simulink model "baseline1"  (R2022b)
settings: Solver=ode4  StartTime=0.0  StopTime=200  FixedStep=1e-3  RelTol=1e-3
undefined symbols (not defined in the file or in its folder): A_do, B_do, c_uf, do_w, f_b, f_max, f_min, F_TOT_MAX, Fz_min, g, G_do, Gamma_mix, Ixx, Iyy, Izz, K_eta, K_omega, K_w, Ka1, Ka2, Ka3, Kgamma, Knu, Kp1, Kp2, Kp3, L, l_axis, l_gain, m, m_p, n_state_axis, p2_bias_acc, p2_h3_s0, p2_ic_do, p2_ic_eso, p2_ic_pos, p2_ic_vel, p2_nd_pos, p2_prm, p2_prm_h3, p2_prm_m3, p2_prm_n6, p2_prm_w, p2_seed_acc, p2_seed_gyro, p2_seed_pos, p2_tau_m, p2_trim_do, p2_trim_eso, p2_trim_ff_v, p2_Ts_att, p2_Ts_pos, p2_var_acc, p2_var_gyro, p2_var_pos, payload_amp, payload_inj_on, payload_K_ratio, payload_model ... (+18)
(part 1 of 3)
settings Model: Creator=Dell  LastModifiedBy=Dell

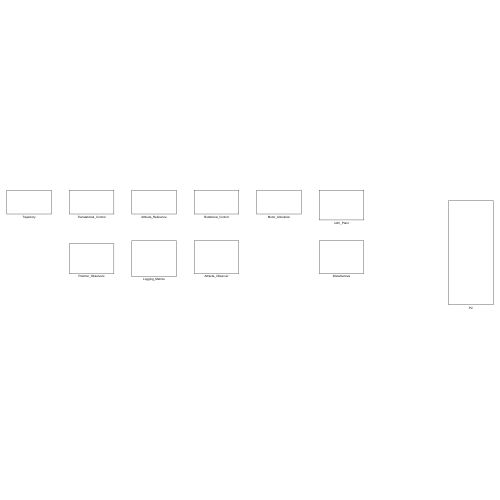
[thumbnail: Simulink's stored preview of the top-level diagram]
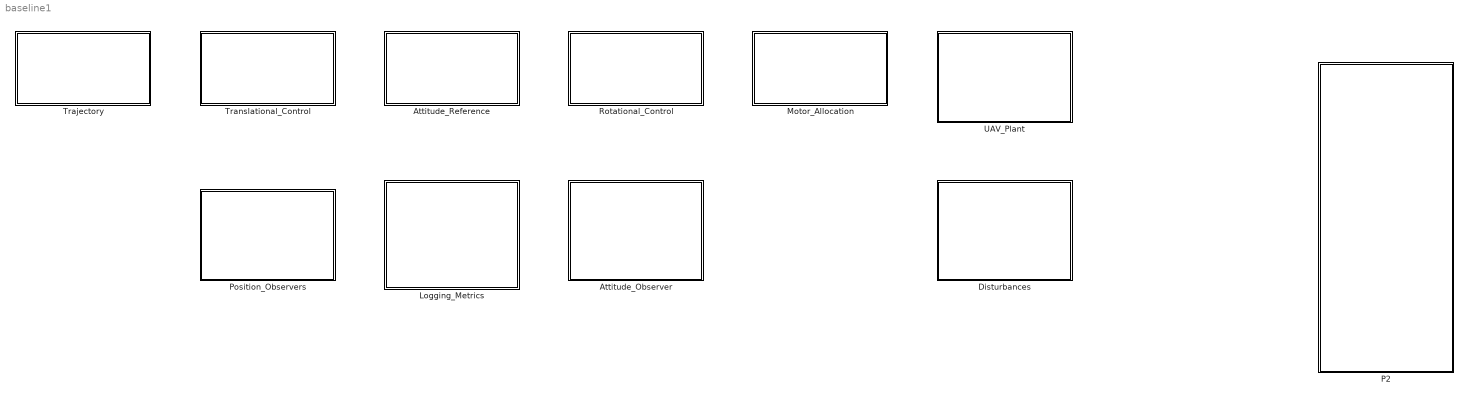
== system baseline1 ==
  Attitude_Observer : Subsystem
  Attitude_Reference : Subsystem
  Disturbances : Subsystem
  Logging_Metrics : Subsystem
  Motor_Allocation : Subsystem
  P2 : Subsystem
  Position_Observers : Subsystem
  Rotational_Control : Subsystem
  Trajectory : Subsystem
  Translational_Control : Subsystem
  UAV_Plant : Subsystem

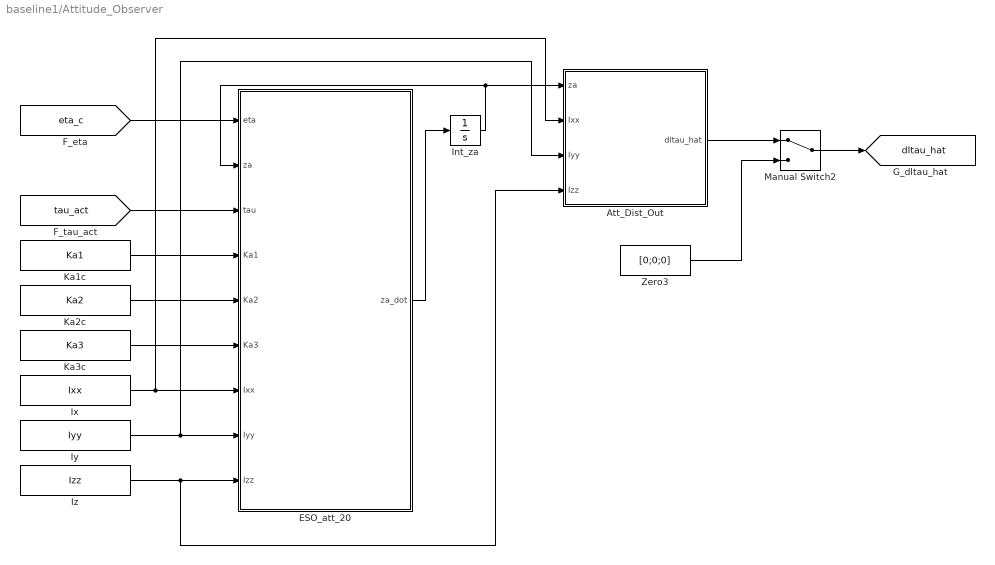
== system baseline1/Attitude_Observer ==
  Att_Dist_Out : MATLAB Function  TreatAsAtomicUnit=on
  ESO_att_20 : MATLAB Function  TreatAsAtomicUnit=on
  Int_za : Integrator
  Ix : Constant  Value=Ixx
  Iy : Constant  Value=Iyy
  Iz : Constant  Value=Izz
  Ka1c : Constant  Value=Ka1
  Ka2c : Constant  Value=Ka2
  Ka3c : Constant  Value=Ka3
  Manual Switch2 : ManualSwitch
  Zero3 : Constant  Value=[0;0;0]
  tag scope: dltau_hat=global
  wires:
  [eta_c] -> ESO_att_20/1(eta)
  [tau_act] -> ESO_att_20/3(tau)
  Ka1c/1 -> ESO_att_20/4(Ka1)
  Ka2c/1 -> ESO_att_20/5(Ka2)
  Ka3c/1 -> ESO_att_20/6(Ka3)
  Ix/1 -> ESO_att_20/7(Ixx), Att_Dist_Out/2(Ixx)
  Iy/1 -> Att_Dist_Out/3(Iyy), ESO_att_20/8(Iyy)
  Iz/1 -> Att_Dist_Out/4(Izz), ESO_att_20/9(Izz)
  ESO_att_20/1(za_dot) -> Int_za/1
  Int_za/1 -> ESO_att_20/2(za), Att_Dist_Out/1(za)
  Att_Dist_Out/1(dltau_hat) -> Manual Switch2/1
  Zero3/1 -> Manual Switch2/2
  Manual Switch2/1 -> [dltau_hat]

== system baseline1/Attitude_Reference ==
  Fzmin : Constant  Value=Fz_min
  P2_FTOT : Constant  Value=F_TOT_MAX
  Thrust_AttRef_16 : MATLAB Function  TreatAsAtomicUnit=on
  psi_d : Constant  Value=0
  tag scope: eta_d=global, fthr=global
  wires:
  [Fcmd_c] -> Thrust_AttRef_16/1(F)
  [eta_c] -> Thrust_AttRef_16/2(eta)
  psi_d/1 -> Thrust_AttRef_16/3(psi_d)
  Fzmin/1 -> Thrust_AttRef_16/4(Fz_min)
  Thrust_AttRef_16/1(f) -> [fthr]
  Thrust_AttRef_16/2(eta_d) -> [eta_d]
  P2_FTOT/1 -> Thrust_AttRef_16/5(F_TOT_MAX)

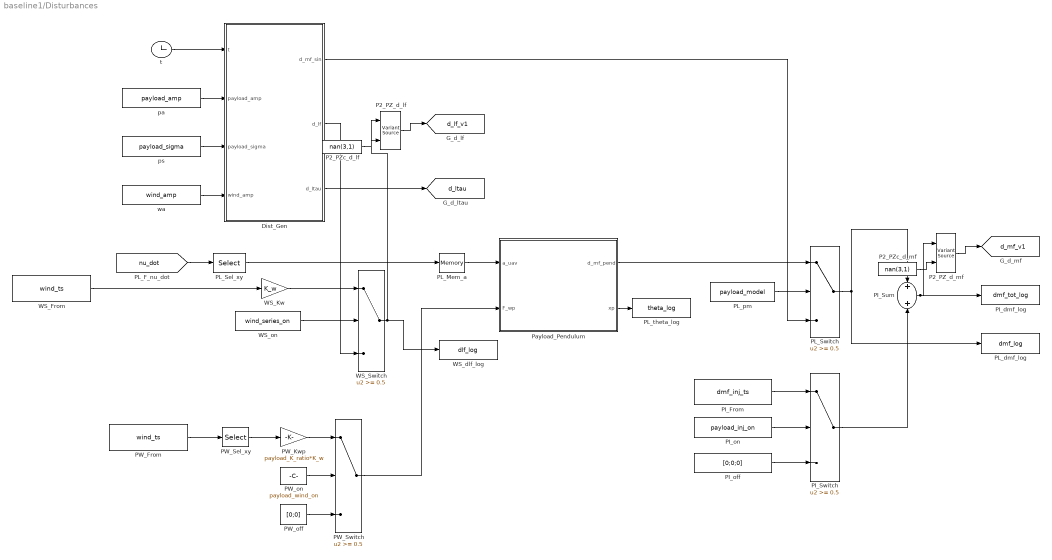
== system baseline1/Disturbances ==
  Dist_Gen : MATLAB Function  TreatAsAtomicUnit=on
  P2_PZ_d_lf : VariantSource
  P2_PZ_d_mf : VariantSource
  P2_PZc_d_lf : Constant  Value=nan(3,1)
  P2_PZc_d_mf : Constant  Value=nan(3,1)
  PI_From : FromWorkspace  VariableName=dmf_inj_ts  OutputAfterFinalValue=Holding final value
  PI_Sum : Sum  Description=PAYLOAD_INJ_ORIG_SRC=PL_Switch/1
  PI_Switch : Switch  Threshold=0.5  SaturateOnIntegerOverflow=off  InputSameDT=off
  PI_dmf_log : ToWorkspace  VariableName=dmf_tot_log  SaveFormat=Structure With Time  SampleTime=-1
  PI_off : Constant  Value=[0;0;0]
  PI_on : Constant  Value=payload_inj_on
  PL_Mem_a : Memory  InitialCondition=[0;0]
  PL_Sel_xy : Selector  InputPortWidth=3  IndexOptions=Index vector (dialog)  Indices=[1 2]  OutputSizes=1
  PL_Switch : Switch  Threshold=0.5  SaturateOnIntegerOverflow=off  InputSameDT=off
  PL_dmf_log : ToWorkspace  VariableName=dmf_log  SaveFormat=Structure With Time  SampleTime=-1
  PL_pm : Constant  Value=payload_model
  PL_theta_log : ToWorkspace  VariableName=theta_log  SaveFormat=Structure With Time  SampleTime=-1
  PW_From : FromWorkspace  VariableName=wind_ts  OutputAfterFinalValue=Holding final value
  PW_Kwp : Gain  Gain=payload_K_ratio*K_w
  PW_Sel_xy : Selector  InputPortWidth=3  IndexOptions=Index vector (dialog)  Indices=[1 2]  OutputSizes=1
  PW_Switch : Switch  Threshold=0.5  SaturateOnIntegerOverflow=off  InputSameDT=off
  PW_off : Constant  Value=[0;0]
  PW_on : Constant  Value=payload_wind_on
  Payload_Pendulum : Subsystem
  WS_From : FromWorkspace  VariableName=wind_ts  OutputAfterFinalValue=Holding final value
  WS_Kw : Gain  Gain=K_w
  WS_Switch : Switch  Description=WIND_SERIES_ORIG_DST=G_d_lf/1  Threshold=0.5  SaturateOnIntegerOverflow=off  InputSameDT=off
  WS_dlf_log : ToWorkspace  VariableName=dlf_log  SaveFormat=Structure With Time  SampleTime=-1
  WS_on : Constant  Value=wind_series_on
  pa : Constant  Value=payload_amp
  ps : Constant  Value=payload_sigma
  t : Clock
  wa : Constant  Value=wind_amp
  tag scope: d_lf_v1=global, d_ltau=global, d_mf_v1=global
  wires:
  t/1 -> Dist_Gen/1(t)
  pa/1 -> Dist_Gen/2(payload_amp)
  ps/1 -> Dist_Gen/3(payload_sigma)
  wa/1 -> Dist_Gen/4(wind_amp)
  Dist_Gen/3(d_ltau) -> [d_ltau]
  WS_From/1 -> WS_Kw/1
  WS_Kw/1 -> WS_Switch/1
  WS_on/1 -> WS_Switch/2
  Dist_Gen/2(d_lf) -> WS_Switch/3
  WS_Switch/1 -> WS_dlf_log/1, P2_PZ_d_lf/1
  [nu_dot] -> PL_Sel_xy/1
  PL_Sel_xy/1 -> PL_Mem_a/1
  PL_Mem_a/1 -> Payload_Pendulum/1(a_uav)
  Payload_Pendulum/1(d_mf_pend) -> PL_Switch/1
  PL_pm/1 -> PL_Switch/2
  Dist_Gen/1(d_mf_sin) -> PL_Switch/3
  PL_Switch/1 -> PI_Sum/1, PL_dmf_log/1
  Payload_Pendulum/2(xp) -> PL_theta_log/1
  PW_From/1 -> PW_Sel_xy/1
  PW_Sel_xy/1 -> PW_Kwp/1
  PW_Kwp/1 -> PW_Switch/1
  PW_on/1 -> PW_Switch/2
  PW_off/1 -> PW_Switch/3
  PW_Switch/1 -> Payload_Pendulum/2(F_wp)
  PI_From/1 -> PI_Switch/1
  PI_on/1 -> PI_Switch/2
  PI_off/1 -> PI_Switch/3
  PI_Switch/1 -> PI_Sum/2
  PI_Sum/1 -> PI_dmf_log/1, P2_PZ_d_mf/1
  P2_PZc_d_mf/1 -> P2_PZ_d_mf/2
  P2_PZ_d_mf/1 -> [d_mf_v1]
  P2_PZc_d_lf/1 -> P2_PZ_d_lf/2
  P2_PZ_d_lf/1 -> [d_lf_v1]

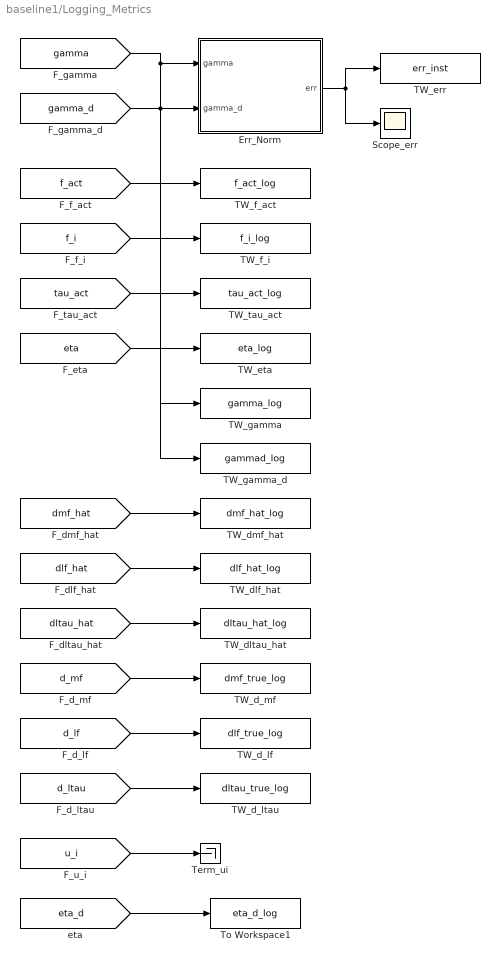
== system baseline1/Logging_Metrics ==
  Err_Norm : MATLAB Function  TreatAsAtomicUnit=on
  Scope_err : Scope
  TW_d_lf : ToWorkspace  VariableName=dlf_true_log  SaveFormat=Structure With Time  SampleTime=-1
  TW_d_ltau : ToWorkspace  VariableName=dltau_true_log  SaveFormat=Structure With Time  SampleTime=-1
  TW_d_mf : ToWorkspace  VariableName=dmf_true_log  SaveFormat=Structure With Time  SampleTime=-1
  TW_dlf_hat : ToWorkspace  VariableName=dlf_hat_log  SaveFormat=Structure With Time  SampleTime=-1
  TW_dltau_hat : ToWorkspace  VariableName=dltau_hat_log  SaveFormat=Structure With Time  SampleTime=-1
  TW_dmf_hat : ToWorkspace  VariableName=dmf_hat_log  SaveFormat=Structure With Time  SampleTime=-1
  TW_err : ToWorkspace  VariableName=err_inst  SaveFormat=Structure With Time  SampleTime=-1
  TW_eta : ToWorkspace  VariableName=eta_log  SaveFormat=Structure With Time  SampleTime=-1
  TW_f_act : ToWorkspace  VariableName=f_act_log  SaveFormat=Structure With Time  SampleTime=-1
  TW_f_i : ToWorkspace  VariableName=f_i_log  SaveFormat=Structure With Time  SampleTime=-1
  TW_gamma : ToWorkspace  VariableName=gamma_log  SaveFormat=Structure With Time  SampleTime=-1
  TW_gamma_d : ToWorkspace  VariableName=gammad_log  SaveFormat=Structure With Time  SampleTime=-1
  TW_tau_act : ToWorkspace  VariableName=tau_act_log  SaveFormat=Structure With Time  SampleTime=-1
  Term_ui : Terminator
  To Workspace1 : ToWorkspace  VariableName=eta_d_log  SampleTime=-1
  wires:
  [gamma] -> Err_Norm/1(gamma), TW_gamma/1
  [gamma_d] -> Err_Norm/2(gamma_d), TW_gamma_d/1
  Err_Norm/1(err) -> TW_err/1, Scope_err/1
  [f_act] -> TW_f_act/1
  [f_i] -> TW_f_i/1
  [tau_act] -> TW_tau_act/1
  [eta] -> TW_eta/1
  [dmf_hat] -> TW_dmf_hat/1
  [dlf_hat] -> TW_dlf_hat/1
  [dltau_hat] -> TW_dltau_hat/1
  [d_mf] -> TW_d_mf/1
  [d_lf] -> TW_d_lf/1
  [d_ltau] -> TW_d_ltau/1
  [u_i] -> Term_ui/1
  [eta_d] -> To Workspace1/1

== system baseline1/Motor_Allocation ==
  Alloc_2_3 : MATLAB Function  TreatAsAtomicUnit=on
  Gm : Constant  Value=Gamma_mix
  cu : Constant  Value=c_uf
  fb : Constant  Value=f_b
  fmn : Constant  Value=f_min
  fmx : Constant  Value=f_max
  ub : Constant  Value=u_b
  tag scope: f_act=global, f_i=global, tau_act=global, u_i=global
  wires:
  [fthr_c] -> Alloc_2_3/1(f_cmd)
  [tau_cmd_c] -> Alloc_2_3/2(tau_cmd)
  Gm/1 -> Alloc_2_3/3(Gamma_mix)
  fmn/1 -> Alloc_2_3/4(f_min)
  fmx/1 -> Alloc_2_3/5(f_max)
  cu/1 -> Alloc_2_3/6(c_uf)
  fb/1 -> Alloc_2_3/7(f_b)
  ub/1 -> Alloc_2_3/8(u_b)
  Alloc_2_3/1(f_act) -> [f_act]
  Alloc_2_3/2(tau_act) -> [tau_act]
  Alloc_2_3/3(f_i) -> [f_i]
  Alloc_2_3/4(u_i) -> [u_i]

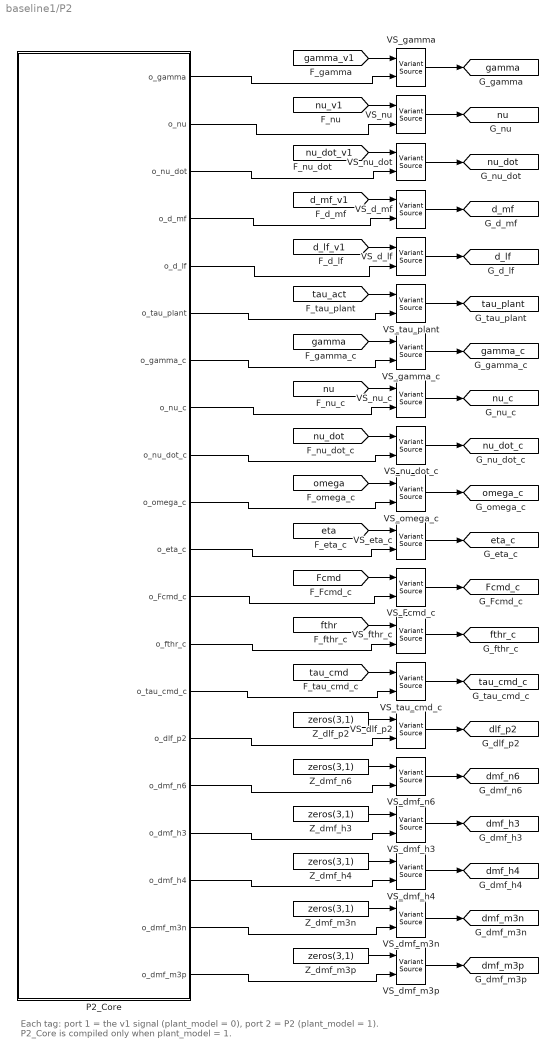
== system baseline1/P2 ==
  note: Each tag: port 1 = the v1 signal (plant_model = 0), port 2 = P2 (plant_model = 1).
      | P2_Core is compiled only when plant_model = 1.
  P2_Core : Subsystem  Variant=on  AllowZeroVariantControls=on  PropagateVariantConditions=on
  VS_Fcmd_c : VariantSource
  VS_d_lf : VariantSource
  VS_d_mf : VariantSource
  VS_dlf_p2 : VariantSource
  VS_dmf_h3 : VariantSource
  VS_dmf_h4 : VariantSource
  VS_dmf_m3n : VariantSource
  VS_dmf_m3p : VariantSource
  VS_dmf_n6 : VariantSource
  VS_eta_c : VariantSource
  VS_fthr_c : VariantSource
  VS_gamma : VariantSource
  VS_gamma_c : VariantSource
  VS_nu : VariantSource
  VS_nu_c : VariantSource
  VS_nu_dot : VariantSource
  VS_nu_dot_c : VariantSource
  VS_omega_c : VariantSource
  VS_tau_cmd_c : VariantSource
  VS_tau_plant : VariantSource
  Z_dlf_p2 : Constant  Value=zeros(3,1)
  Z_dmf_h3 : Constant  Value=zeros(3,1)
  Z_dmf_h4 : Constant  Value=zeros(3,1)
  Z_dmf_m3n : Constant  Value=zeros(3,1)
  Z_dmf_m3p : Constant  Value=zeros(3,1)
  Z_dmf_n6 : Constant  Value=zeros(3,1)
  tag scope: Fcmd_c=global, d_lf=global, d_mf=global, dlf_p2=global, dmf_h3=global, dmf_h4=global, dmf_m3n=global, dmf_m3p=global, dmf_n6=global, eta_c=global, fthr_c=global, gamma=global, gamma_c=global, nu=global, nu_c=global, nu_dot=global, nu_dot_c=global, omega_c=global, tau_cmd_c=global, tau_plant=global
  wires:
  VS_Fcmd_c/1 -> [Fcmd_c]
  VS_d_lf/1 -> [d_lf]
  VS_d_mf/1 -> [d_mf]
  VS_dlf_p2/1 -> [dlf_p2]
  VS_dmf_h3/1 -> [dmf_h3]
  VS_dmf_h4/1 -> [dmf_h4]
  VS_dmf_m3n/1 -> [dmf_m3n]
  VS_dmf_m3p/1 -> [dmf_m3p]
  VS_dmf_n6/1 -> [dmf_n6]
  VS_eta_c/1 -> [eta_c]
  VS_fthr_c/1 -> [fthr_c]
  VS_gamma/1 -> [gamma]
  VS_gamma_c/1 -> [gamma_c]
  VS_nu/1 -> [nu]
  VS_nu_c/1 -> [nu_c]
  VS_nu_dot/1 -> [nu_dot]
  VS_nu_dot_c/1 -> [nu_dot_c]
  VS_omega_c/1 -> [omega_c]
  VS_tau_cmd_c/1 -> [tau_cmd_c]
  VS_tau_plant/1 -> [tau_plant]
  [Fcmd] -> VS_Fcmd_c/1
  P2_Core/12(o_Fcmd_c) -> VS_Fcmd_c/2
  [d_lf_v1] -> VS_d_lf/1
  P2_Core/5(o_d_lf) -> VS_d_lf/2
  [d_mf_v1] -> VS_d_mf/1
  P2_Core/4(o_d_mf) -> VS_d_mf/2
  Z_dlf_p2/1 -> VS_dlf_p2/1
  P2_Core/15(o_dlf_p2) -> VS_dlf_p2/2
  Z_dmf_h3/1 -> VS_dmf_h3/1
  P2_Core/17(o_dmf_h3) -> VS_dmf_h3/2
  Z_dmf_h4/1 -> VS_dmf_h4/1
  P2_Core/18(o_dmf_h4) -> VS_dmf_h4/2
  Z_dmf_m3n/1 -> VS_dmf_m3n/1
  P2_Core/19(o_dmf_m3n) -> VS_dmf_m3n/2
  Z_dmf_m3p/1 -> VS_dmf_m3p/1
  P2_Core/20(o_dmf_m3p) -> VS_dmf_m3p/2
  Z_dmf_n6/1 -> VS_dmf_n6/1
  P2_Core/16(o_dmf_n6) -> VS_dmf_n6/2
  [eta] -> VS_eta_c/1
  P2_Core/11(o_eta_c) -> VS_eta_c/2
  [fthr] -> VS_fthr_c/1
  P2_Core/13(o_fthr_c) -> VS_fthr_c/2
  [gamma_v1] -> VS_gamma/1
  P2_Core/1(o_gamma) -> VS_gamma/2
  [gamma] -> VS_gamma_c/1
  P2_Core/7(o_gamma_c) -> VS_gamma_c/2
  [nu_v1] -> VS_nu/1
  P2_Core/2(o_nu) -> VS_nu/2
  [nu] -> VS_nu_c/1
  P2_Core/8(o_nu_c) -> VS_nu_c/2
  [nu_dot_v1] -> VS_nu_dot/1
  P2_Core/3(o_nu_dot) -> VS_nu_dot/2
  [nu_dot] -> VS_nu_dot_c/1
  P2_Core/9(o_nu_dot_c) -> VS_nu_dot_c/2
  [omega] -> VS_omega_c/1
  P2_Core/10(o_omega_c) -> VS_omega_c/2
  [tau_cmd] -> VS_tau_cmd_c/1
  P2_Core/14(o_tau_cmd_c) -> VS_tau_cmd_c/2
  [tau_act] -> VS_tau_plant/1
  P2_Core/6(o_tau_plant) -> VS_tau_plant/2

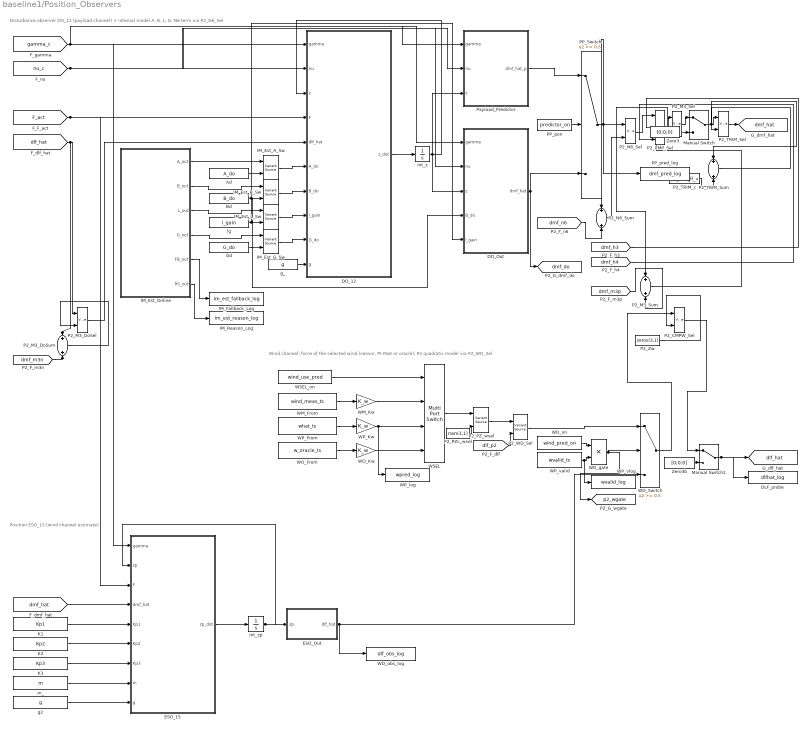
== system baseline1/Position_Observers ==
  note: Disturbance observer DO_12 (payload channel) + internal model A, B, L, G; N6 term via P2_N6_Sel
  note: Wind channel: force of the selected wind (sensor, PI-MoE or oracle); P2 quadratic model via P2_WD_Sel
  note: Position ESO_15 (wind channel estimate)
  Ad : Constant  Value=A_do
  Bd : Constant  Value=B_do
  DLF_probe : ToWorkspace  VariableName=dlfhat_log  SaveFormat=Structure With Time  SampleTime=-1
  DO_12 : MATLAB Function  TreatAsAtomicUnit=on
  DO_Out : MATLAB Function  TreatAsAtomicUnit=on
  ESO_15 : MATLAB Function  TreatAsAtomicUnit=on
  ESO_Out : MATLAB Function  TreatAsAtomicUnit=on
  Gd : Constant  Value=G_do
  IM_Est_A_Sw : VariantSource
  IM_Est_B_Sw : VariantSource
  IM_Est_G_Sw : VariantSource
  IM_Est_L_Sw : VariantSource
  IM_Est_Online : Subsystem
  IM_Fallback_Log : ToWorkspace  VariableName=im_est_fallback_log  SaveFormat=Structure With Time  SampleTime=-1
  IM_Reason_Log : ToWorkspace  VariableName=im_est_reason_log  SaveFormat=Structure With Time  SampleTime=-1
  Int_z : Integrator  InitialCondition=p2_ic_do(l_gain, R_traj, z0_hover, w_traj, plant_model, p2_trim_do, p2_ic_pos, p2_ic_vel)
  Int_zp : Integrator  InitialCondition=p2_ic_eso(R_traj, z0_hover, w_traj, plant_model, p2_trim_eso, p2_ic_pos, p2_ic_vel)
  K1 : Constant  Value=Kp1
  K2 : Constant  Value=Kp2
  K3 : Constant  Value=Kp3
  Manual Switch : ManualSwitch
  Manual Switch1 : ManualSwitch
  P2_CMPW_Sel : VariantSource
  P2_CMP_Sel : VariantSource
  P2_M3_DoSel : VariantSource
  P2_M3_DoSum : Sum
  P2_M3_Sel : VariantSource
  P2_M3_Sum : Sum
  P2_N6_Sel : VariantSource
  P2_N6_Sum : Sum
  P2_PZ_wsel : VariantSource
  P2_PZc_wsel : Constant  Value=nan(3,1)
  P2_TRIM_Sel : VariantSource
  P2_TRIM_Sum : Sum
  P2_TRIM_c : Constant  Value=p2_trim_ff_v
  P2_WD_Sel : VariantSource
  P2_Zw : Constant  Value=zeros(3,1)
  PP_Switch : Switch  Threshold=0.5  SaturateOnIntegerOverflow=off  InputSameDT=off
  PP_pon : Constant  Value=predictor_on
  PP_pred_log : ToWorkspace  VariableName=dmf_pred_log  SaveFormat=Structure With Time  SampleTime=-1
  Payload_Predictor : Subsystem
  WD_Switch : Switch  Description=PA_MOBADC_ORIG_SRC=ESO_Out/1  Threshold=0.5  SaturateOnIntegerOverflow=off  InputSameDT=off
  WD_gate : Product
  WD_obs_log : ToWorkspace  VariableName=dlf_obs_log  SaveFormat=Structure With Time  SampleTime=-1
  WD_on : Constant  Value=wind_pred_on
  WM_From : FromWorkspace  VariableName=wind_meas_ts  Interpolate=off  OutputAfterFinalValue=Holding final value
  WM_Kw : Gain  Gain=K_w
  WO_From : FromWorkspace  VariableName=w_oracle_ts  Interpolate=off  OutputAfterFinalValue=Holding final value
  WO_Kw : Gain  Gain=K_w
  WP_From : FromWorkspace  VariableName=what_ts  Interpolate=off  OutputAfterFinalValue=Holding final value
  WP_Kw : Gain  Gain=K_w
  WP_log : ToWorkspace  VariableName=wpred_log  SaveFormat=Structure With Time  SampleTime=-1
  WP_valid : FromWorkspace  VariableName=wvalid_ts  Interpolate=off  OutputAfterFinalValue=Holding final value
  WP_vlog : ToWorkspace  VariableName=wvalid_log  SaveFormat=Structure With Time  SampleTime=-1
  WSEL : MultiPortSwitch  DataPortOrder=Zero-based contiguous  zeroidx=on  SaturateOnIntegerOverflow=off  InputSameDT=off
  WSEL_on : Constant  Value=wind_use_pred
  Zero3 : Constant  Value=[0;0;0]
  Zero3b : Constant  Value=[0;0;0]
  g2 : Constant  Value=g
  g_ : Constant  Value=g
  lg : Constant  Value=l_gain
  m_ : Constant  Value=m
  tag scope: dlf_hat=global, dmf_do=global, dmf_hat=global, p2_wgate=global
  wires:
  Manual Switch1/1 -> DLF_probe/1, [dlf_hat]
  [gamma_c] -> DO_12/1(gamma), DO_Out/1(gamma), ESO_15/1(gamma), Payload_Predictor/1(gamma)
  [nu_c] -> DO_12/2(nu), DO_Out/2(nu), Payload_Predictor/2(nu)
  Int_z/1 -> DO_12/3(z), DO_Out/3(z), Payload_Predictor/3(z)
  [F_act] -> DO_12/4(F), ESO_15/3(F)
  P2_M3_DoSel/1 -> DO_12/5(dlf_hat)
  IM_Est_A_Sw/1 -> DO_12/6(A_do)
  IM_Est_B_Sw/1 -> DO_12/7(B_do)
  IM_Est_L_Sw/1 -> DO_12/8(l_gain)
  IM_Est_G_Sw/1 -> DO_12/9(G_do)
  g_/1 -> DO_12/10(g)
  Bd/1 -> DO_Out/4(B_do), IM_Est_B_Sw/2
  lg/1 -> DO_Out/5(l_gain), IM_Est_L_Sw/2
  Int_zp/1 -> ESO_15/2(zp), ESO_Out/1(zp)
  [dmf_hat] -> ESO_15/4(dmf_hat)
  K1/1 -> ESO_15/5(Kp1)
  K2/1 -> ESO_15/6(Kp2)
  K3/1 -> ESO_15/7(Kp3)
  m_/1 -> ESO_15/8(m)
  g2/1 -> ESO_15/9(g)
  P2_TRIM_Sel/1 -> [dmf_hat]
  IM_Est_Online/1(A_out) -> IM_Est_A_Sw/1
  Ad/1 -> IM_Est_A_Sw/2
  IM_Est_Online/2(B_out) -> IM_Est_B_Sw/1
  IM_Est_Online/4(G_out) -> IM_Est_G_Sw/1
  Gd/1 -> IM_Est_G_Sw/2
  IM_Est_Online/3(L_out) -> IM_Est_L_Sw/1
  IM_Est_Online/5(FB_out) -> IM_Fallback_Log/1
  IM_Est_Online/6(RS_out) -> IM_Reason_Log/1
  DO_12/1(z_dot) -> Int_z/1
  ESO_15/1(zp_dot) -> Int_zp/1
  P2_M3_Sel/1 -> Manual Switch/1
  Zero3/1 -> Manual Switch/2
  P2_CMPW_Sel/1 -> Manual Switch1/1
  Zero3b/1 -> Manual Switch1/2
  WD_Switch/1 -> P2_CMPW_Sel/1
  P2_Zw/1 -> P2_CMPW_Sel/2
  P2_N6_Sel/1 -> P2_CMP_Sel/1
  [dmf_h3] -> P2_CMP_Sel/2
  [dmf_h4] -> P2_CMP_Sel/3
  DO_Out/1(dmf_hat) -> [dmf_do], PP_Switch/3
  WD_gate/1 -> [p2_wgate], WD_Switch/2
  [dlf_hat] -> P2_M3_DoSel/1, P2_M3_DoSum/1
  P2_M3_DoSum/1 -> P2_M3_DoSel/2
  [dmf_m3n] -> P2_M3_DoSum/2
  P2_CMP_Sel/1 -> P2_M3_Sel/1, P2_M3_Sum/1
  P2_M3_Sum/1 -> P2_M3_Sel/2
  [dmf_m3p] -> P2_M3_Sum/2
  PP_Switch/1 -> P2_N6_Sel/1, P2_N6_Sum/1, PP_pred_log/1
  P2_N6_Sum/1 -> P2_N6_Sel/2
  [dmf_n6] -> P2_N6_Sum/2
  WSEL/1 -> P2_PZ_wsel/1
  P2_PZc_wsel/1 -> P2_PZ_wsel/2
  Manual Switch/1 -> P2_TRIM_Sel/1, P2_TRIM_Sum/1
  P2_TRIM_Sum/1 -> P2_TRIM_Sel/2
  P2_TRIM_c/1 -> P2_TRIM_Sum/2
  P2_PZ_wsel/1 -> P2_WD_Sel/1
  [dlf_p2] -> P2_WD_Sel/2
  Payload_Predictor/1(dmf_hat_p) -> PP_Switch/1
  PP_pon/1 -> PP_Switch/2
  P2_WD_Sel/1 -> WD_Switch/1
  ESO_Out/1(dlf_hat) -> WD_Switch/3, WD_obs_log/1
  WD_on/1 -> WD_gate/1
  WP_valid/1 -> WD_gate/2, WP_vlog/1
  WM_From/1 -> WM_Kw/1
  WO_From/1 -> WO_Kw/1
  WP_From/1 -> WP_Kw/1
  WP_Kw/1 -> WP_log/1, WSEL/3
  WSEL_on/1 -> WSEL/1
  WM_Kw/1 -> WSEL/2
  WO_Kw/1 -> WSEL/4

== system baseline1/Rotational_Control ==
  Att_Ctrl_18 : MATLAB Function  TreatAsAtomicUnit=on
  Keta : Constant  Value=K_eta
  Kom : Constant  Value=K_omega
  tag scope: tau_cmd=global
  wires:
  [eta_d] -> Att_Ctrl_18/1(eta_d)
  [eta_c] -> Att_Ctrl_18/2(eta)
  [omega_c] -> Att_Ctrl_18/3(omega)
  [dltau_hat] -> Att_Ctrl_18/4(dltau_hat)
  Keta/1 -> Att_Ctrl_18/5(K_eta)
  Kom/1 -> Att_Ctrl_18/6(K_omega)
  Att_Ctrl_18/1(tau_cmd) -> [tau_cmd]

== system baseline1/Trajectory ==
  R : Constant  Value=R_traj
  TR_tauprev : Constant  Value=tau_prev
  TR_trajpar : Constant  Value=traj_par
  TR_trajtype : Constant  Value=traj_type
  Traj_Ref : MATLAB Function  TreatAsAtomicUnit=on
  t : Clock
  w : Constant  Value=w_traj
  z0 : Constant  Value=z0_hover
  tag scope: acc_d=global, gamma_d=global, nu_d=global
  wires:
  t/1 -> Traj_Ref/1(t)
  R/1 -> Traj_Ref/2(R)
  w/1 -> Traj_Ref/3(w)
  z0/1 -> Traj_Ref/4(z0)
  Traj_Ref/1(gamma_d) -> [gamma_d]
  Traj_Ref/2(nu_d) -> [nu_d]
  Traj_Ref/3(acc_d) -> [acc_d]
  TR_tauprev/1 -> Traj_Ref/5(tau_prev)
  TR_trajtype/1 -> Traj_Ref/6(traj_type)
  TR_trajpar/1 -> Traj_Ref/7(traj_par)

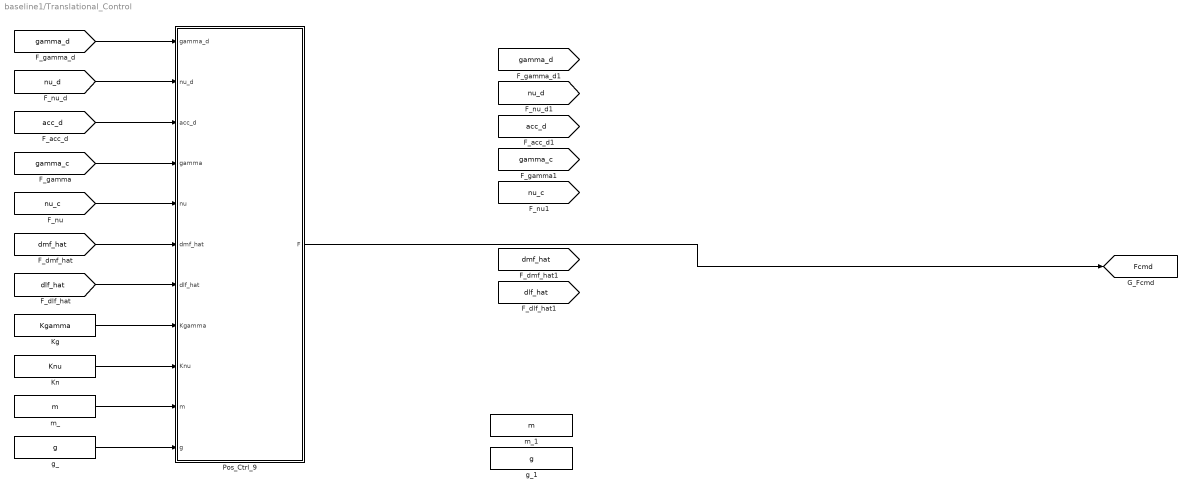
== system baseline1/Translational_Control ==
  Kg : Constant  Value=Kgamma
  Kn : Constant  Value=Knu
  Pos_Ctrl_9 : MATLAB Function  TreatAsAtomicUnit=on
  g_ : Constant  Value=g
  g_1 : Constant  Value=g
  m_ : Constant  Value=m
  m_1 : Constant  Value=m
  tag scope: Fcmd=global
  wires:
  [gamma_d] -> Pos_Ctrl_9/1(gamma_d)
  [nu_d] -> Pos_Ctrl_9/2(nu_d)
  [acc_d] -> Pos_Ctrl_9/3(acc_d)
  [gamma_c] -> Pos_Ctrl_9/4(gamma)
  [nu_c] -> Pos_Ctrl_9/5(nu)
  [dmf_hat] -> Pos_Ctrl_9/6(dmf_hat)
  [dlf_hat] -> Pos_Ctrl_9/7(dlf_hat)
  Kg/1 -> Pos_Ctrl_9/8(Kgamma)
  Kn/1 -> Pos_Ctrl_9/9(Knu)
  m_/1 -> Pos_Ctrl_9/10(m)
  g_/1 -> Pos_Ctrl_9/11(g)
  Pos_Ctrl_9/1(F) -> [Fcmd]

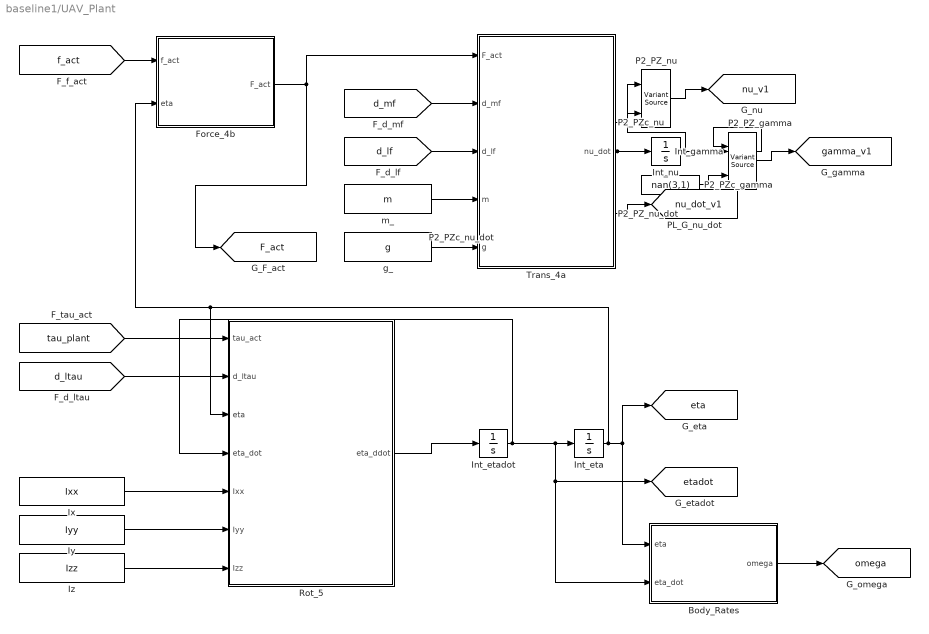
== system baseline1/UAV_Plant ==
  Body_Rates : MATLAB Function  TreatAsAtomicUnit=on
  Force_4b : MATLAB Function  TreatAsAtomicUnit=on
  Int_eta : Integrator
  Int_etadot : Integrator
  Int_gamma : Integrator  InitialCondition=[R_traj; 0; z0_hover]
  Int_nu : Integrator  InitialCondition=[0; R_traj*w_traj; 0]
  Ix : Constant  Value=Ixx
  Iy : Constant  Value=Iyy
  Iz : Constant  Value=Izz
  P2_PZ_gamma : VariantSource
  P2_PZ_nu : VariantSource
  P2_PZ_nu_dot : VariantSource
  P2_PZc_gamma : Constant  Value=nan(3,1)
  P2_PZc_nu : Constant  Value=nan(3,1)
  P2_PZc_nu_dot : Constant  Value=nan(3,1)
  Rot_5 : MATLAB Function  TreatAsAtomicUnit=on
  Trans_4a : MATLAB Function  TreatAsAtomicUnit=on
  g_ : Constant  Value=g
  m_ : Constant  Value=m
  tag scope: F_act=global, eta=global, etadot=global, gamma_v1=global, nu_dot_v1=global, nu_v1=global, omega=global
  wires:
  [f_act] -> Force_4b/1(f_act)
  Force_4b/1(F_act) -> Trans_4a/1(F_act), [F_act]
  [d_mf] -> Trans_4a/2(d_mf)
  [d_lf] -> Trans_4a/3(d_lf)
  m_/1 -> Trans_4a/4(m)
  g_/1 -> Trans_4a/5(g)
  Trans_4a/1(nu_dot) -> Int_nu/1, P2_PZ_nu_dot/1
  Int_nu/1 -> Int_gamma/1, P2_PZ_nu/1
  [tau_plant] -> Rot_5/1(tau_act)
  [d_ltau] -> Rot_5/2(d_ltau)
  Ix/1 -> Rot_5/5(Ixx)
  Iy/1 -> Rot_5/6(Iyy)
  Iz/1 -> Rot_5/7(Izz)
  Rot_5/1(eta_ddot) -> Int_etadot/1
  Int_etadot/1 -> [etadot], Body_Rates/2(eta_dot), Int_eta/1, Rot_5/4(eta_dot)
  Int_eta/1 -> [eta], Body_Rates/1(eta), Rot_5/3(eta), Force_4b/2(eta)
  Body_Rates/1(omega) -> [omega]
  Int_gamma/1 -> P2_PZ_gamma/1
  P2_PZc_gamma/1 -> P2_PZ_gamma/2
  P2_PZ_gamma/1 -> [gamma_v1]
  P2_PZc_nu/1 -> P2_PZ_nu/2
  P2_PZ_nu/1 -> [nu_v1]
  P2_PZc_nu_dot/1 -> P2_PZ_nu_dot/2
  P2_PZ_nu_dot/1 -> [nu_dot_v1]

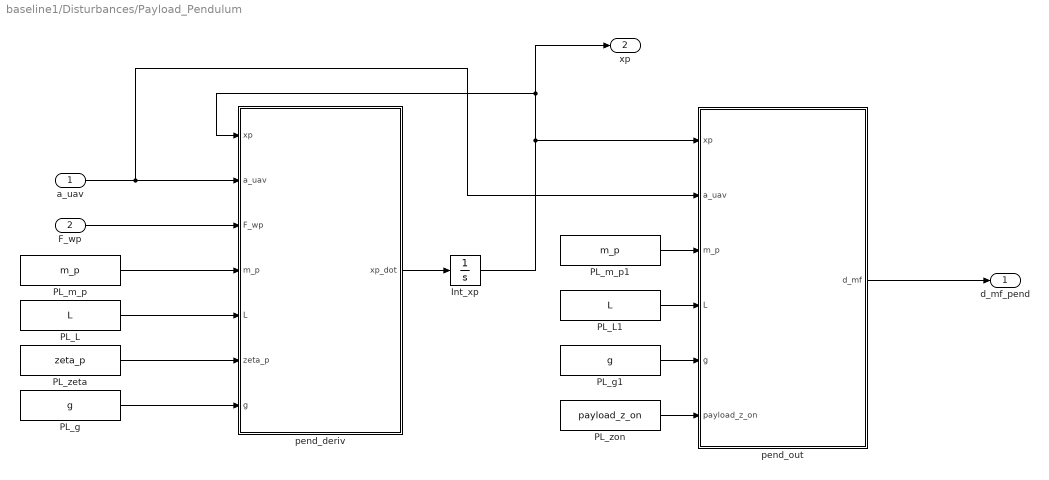
== system baseline1/Disturbances/Payload_Pendulum ==
  a_uav : Inport
  F_wp : Inport  Port=2
  Int_xp : Integrator  InitialCondition=[0;0;0;0]
  PL_L : Constant  Value=L
  PL_L1 : Constant  Value=L
  PL_g : Constant  Value=g
  PL_g1 : Constant  Value=g
  PL_m_p : Constant  Value=m_p
  PL_m_p1 : Constant  Value=m_p
  PL_zeta : Constant  Value=zeta_p
  PL_zon : Constant  Value=payload_z_on
  pend_deriv : MATLAB Function  TreatAsAtomicUnit=on
  pend_out : MATLAB Function  TreatAsAtomicUnit=on
  d_mf_pend : Outport
  xp : Outport  Port=2
  wires:
  Int_xp/1 -> pend_deriv/1(xp), xp/1, pend_out/1(xp)
  a_uav/1 -> pend_out/2(a_uav), pend_deriv/2(a_uav)
  F_wp/1 -> pend_deriv/3(F_wp)
  PL_m_p/1 -> pend_deriv/4(m_p)
  PL_L/1 -> pend_deriv/5(L)
  PL_zeta/1 -> pend_deriv/6(zeta_p)
  PL_g/1 -> pend_deriv/7(g)
  pend_deriv/1(xp_dot) -> Int_xp/1
  PL_zon/1 -> pend_out/6(payload_z_on)
  pend_out/1(d_mf) -> d_mf_pend/1
  PL_m_p1/1 -> pend_out/3(m_p)
  PL_L1/1 -> pend_out/4(L)
  PL_g1/1 -> pend_out/5(g)

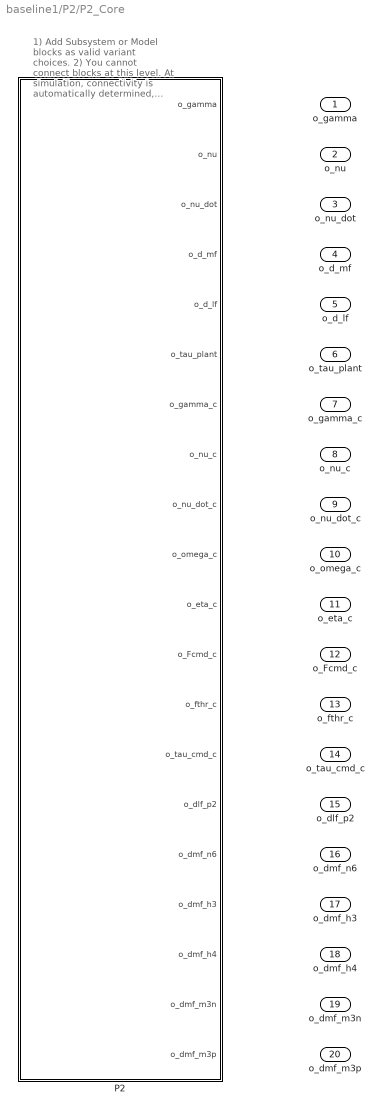
== system baseline1/P2/P2_Core ==
  note: 1) Add Subsystem or Model blocks as valid variant choices.
      | 2) You cannot connect blocks at this level. At simulation, connectivity is automatically
      | determined, based on the active variant and port name matching.
  P2 : Subsystem  VariantControl=plant_model==1
  o_gamma : Outport
  o_nu : Outport  Port=2
  o_nu_dot : Outport  Port=3
  o_d_mf : Outport  Port=4
  o_d_lf : Outport  Port=5
  o_tau_plant : Outport  Port=6
  o_gamma_c : Outport  Port=7
  o_nu_c : Outport  Port=8
  o_nu_dot_c : Outport  Port=9
  o_omega_c : Outport  Port=10
  o_eta_c : Outport  Port=11
  o_Fcmd_c : Outport  Port=12
  o_fthr_c : Outport  Port=13
  o_tau_cmd_c : Outport  Port=14
  o_dlf_p2 : Outport  Port=15
  o_dmf_n6 : Outport  Port=16
  o_dmf_h3 : Outport  Port=17
  o_dmf_h4 : Outport  Port=18
  o_dmf_m3n : Outport  Port=19
  o_dmf_m3p : Outport  Port=20

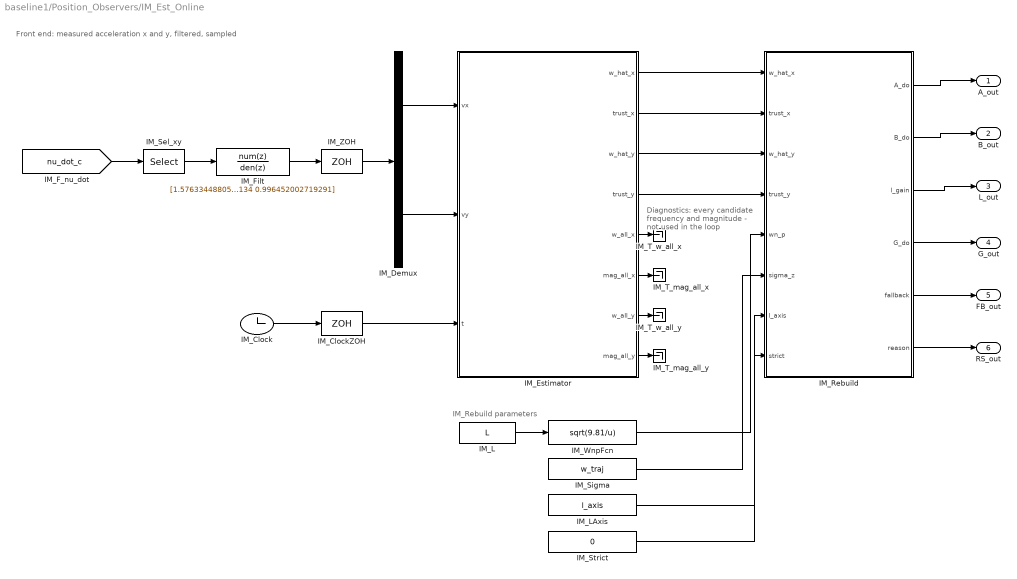
== system baseline1/Position_Observers/IM_Est_Online ==
  note: Front end: measured acceleration x and y, filtered, sampled
  note: Diagnostics: every candidate frequency and magnitude - not used in the loop
  note: IM_Rebuild parameters
  IM_Clock : Clock
  IM_ClockZOH : ZeroOrderHold
  IM_Demux : Demux  Outputs=2
  IM_Estimator : MATLAB Function  TreatAsAtomicUnit=on
  IM_Filt : DiscreteFilter  Numerator=[1.57633448805864e-06 3.15266897611727e-06 1.57633448805864e-06]  Denominator=[1 -1.99644569738134 0.996452002719291]  SampleTime=0.001
  IM_L : Constant  Value=L
  IM_LAxis : Constant  Value=l_axis
  IM_Rebuild : MATLAB Function  TreatAsAtomicUnit=on
  IM_Sel_xy : Selector  InputPortWidth=3  IndexOptions=Index vector (dialog)  Indices=[1 2]  OutputSizes=1
  IM_Sigma : Constant  Value=w_traj
  IM_Strict : Constant  Value=0
  IM_T_mag_all_x : Terminator
  IM_T_mag_all_y : Terminator
  IM_T_w_all_x : Terminator
  IM_T_w_all_y : Terminator
  IM_WnpFcn : Fcn  Expr=sqrt(9.81/u)
  IM_ZOH : ZeroOrderHold
  A_out : Outport
  B_out : Outport  Port=2
  L_out : Outport  Port=3
  G_out : Outport  Port=4
  FB_out : Outport  Port=5
  RS_out : Outport  Port=6
  wires:
  IM_Clock/1 -> IM_ClockZOH/1
  IM_ZOH/1 -> IM_Demux/1
  IM_Demux/1 -> IM_Estimator/1(vx)
  IM_Demux/2 -> IM_Estimator/2(vy)
  IM_ClockZOH/1 -> IM_Estimator/3(t)
  IM_Sel_xy/1 -> IM_Filt/1
  IM_Estimator/1(w_hat_x) -> IM_Rebuild/1(w_hat_x)
  IM_Estimator/2(trust_x) -> IM_Rebuild/2(trust_x)
  IM_Estimator/3(w_hat_y) -> IM_Rebuild/3(w_hat_y)
  IM_Estimator/4(trust_y) -> IM_Rebuild/4(trust_y)
  IM_WnpFcn/1 -> IM_Rebuild/5(wn_p)
  IM_Sigma/1 -> IM_Rebuild/6(sigma_z)
  IM_LAxis/1 -> IM_Rebuild/7(l_axis)
  IM_Strict/1 -> IM_Rebuild/8(strict)
  [nu_dot_c] -> IM_Sel_xy/1
  IM_Estimator/6(mag_all_x) -> IM_T_mag_all_x/1
  IM_Estimator/8(mag_all_y) -> IM_T_mag_all_y/1
  IM_Estimator/5(w_all_x) -> IM_T_w_all_x/1
  IM_Estimator/7(w_all_y) -> IM_T_w_all_y/1
  IM_L/1 -> IM_WnpFcn/1
  IM_Filt/1 -> IM_ZOH/1
  IM_Rebuild/1(A_do) -> A_out/1
  IM_Rebuild/2(B_do) -> B_out/1
  IM_Rebuild/3(l_gain) -> L_out/1
  IM_Rebuild/4(G_do) -> G_out/1
  IM_Rebuild/5(fallback) -> FB_out/1
  IM_Rebuild/6(reason) -> RS_out/1

== system baseline1/Position_Observers/Payload_Predictor ==
  gamma : Inport
  nu : Inport  Port=2
  z : Inport  Port=3
  PP_lg : Constant  Value=l_gain
  PP_nax : Constant  Value=n_state_axis
  PP_sigma : Constant  Value=do_w
  PP_tau : Constant  Value=tau_pred
  pred_fcn : MATLAB Function  TreatAsAtomicUnit=on
  dmf_hat_p : Outport
  wires:
  gamma/1 -> pred_fcn/1(gamma)
  nu/1 -> pred_fcn/2(nu)
  z/1 -> pred_fcn/3(z)
  PP_lg/1 -> pred_fcn/4(l_gain)
  PP_sigma/1 -> pred_fcn/5(do_w)
  PP_nax/1 -> pred_fcn/6(n_state_axis)
  PP_tau/1 -> pred_fcn/7(tau_pred)
  pred_fcn/1(dmf_hat_p) -> dmf_hat_p/1

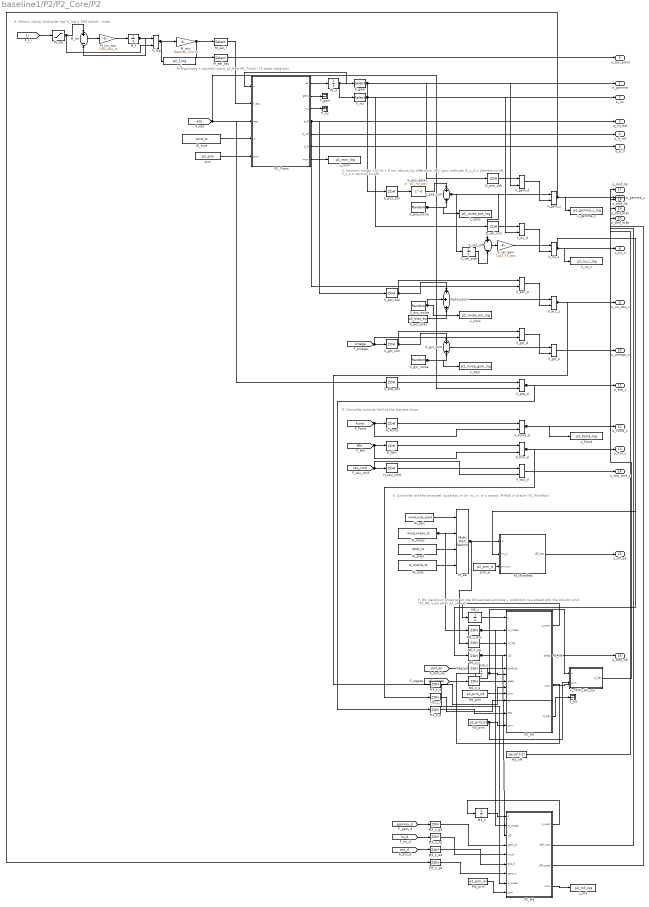
== system baseline1/P2/P2_Core/P2 ==
  note: A. Motors: clamp, first-order lag (V_lag = GD3 switch), mixer
  note: B. Rigid body + payload: plant_p2_free (P2_Trans), 12-state integrator
  note: C. Sensors: mocap 125 Hz + 8 ms, velocity by difference, IMU, gyro, attitude (V_x_d = discrete on-off, V_x_s = sensors on-off)
  note: D. Controller outputs held by the discrete loops
  note: E. Controller wind-force model: quadratic in (w - nu_c), w = sensor, PI-MoE or oracle (P2_WindHat)
  note: F. N6: pendulum observer on the DO payload estimate + prediction tau ahead with the column wind (P2_N6, used when p2_n6 = 1)
  D_pos_zoh : ZeroOrderHold  SampleTime=p2_Ts_pos
  D_vel_zoh : ZeroOrderHold  SampleTime=p2_Ts_pos
  H3_prm : Constant  Value=p2_prm_h3
  H3_s : UnitDelay  InitialCondition=p2_h3_s0  SampleTime=p2_Ts_att  HasFrameUpgradeWarning=on
  H3_z_a : ZeroOrderHold  SampleTime=p2_Ts_att
  H3_z_e : ZeroOrderHold  SampleTime=p2_Ts_att
  H3_z_f : ZeroOrderHold  SampleTime=p2_Ts_att
  H4_off : Constant  Value=zeros(3,1)
  H_Fcmd : ZeroOrderHold  SampleTime=p2_Ts_pos
  H_fthr : ZeroOrderHold  SampleTime=p2_Ts_att
  H_tau_cmd : ZeroOrderHold  SampleTime=p2_Ts_att
  L_Fcmd : ToWorkspace  VariableName=p2_Fcmd_log  SaveFormat=Structure With Time  SampleTime=-1
  L_f : ToWorkspace  VariableName=p2_f_log  SaveFormat=Structure With Time  SampleTime=-1
      settings: Decimation=p2_log_dec
  L_gamma_c : ToWorkspace  VariableName=p2_gamma_c_log  SaveFormat=Structure With Time  SampleTime=-1
  L_m3 : ToWorkspace  VariableName=p2_m3_log  SaveFormat=Structure With Time  SampleTime=-1
      settings: Decimation=p2_log_dec
  L_mon : ToWorkspace  VariableName=p2_mon_log  SaveFormat=Structure With Time  SampleTime=-1
  L_n6 : ToWorkspace  VariableName=p2_n6_log  SaveFormat=Structure With Time  SampleTime=-1
      settings: Decimation=p2_log_dec
  L_nacc : ToWorkspace  VariableName=p2_noise_acc_log  SaveFormat=Structure With Time  SampleTime=-1
  L_ngyr : ToWorkspace  VariableName=p2_noise_gyro_log  SaveFormat=Structure With Time  SampleTime=-1
  L_npos : ToWorkspace  VariableName=p2_noise_pos_log  SaveFormat=Structure With Time  SampleTime=-1
  L_nu_c : ToWorkspace  VariableName=p2_nu_c_log  SaveFormat=Structure With Time  SampleTime=-1
  M3_prm : Constant  Value=p2_prm_m3
  M3_s : UnitDelay  InitialCondition=zeros(4,1)  SampleTime=p2_Ts_att  HasFrameUpgradeWarning=on
  M3_z_ad : ZeroOrderHold  SampleTime=p2_Ts_att
  M3_z_gc : ZeroOrderHold  SampleTime=p2_Ts_att
  M3_z_gd : ZeroOrderHold  SampleTime=p2_Ts_att
  M3_z_nd : ZeroOrderHold  SampleTime=p2_Ts_att
  M_err : Sum  Inputs=+-
  M_f : Integrator  InitialCondition=(m + m_p)*g/4*ones(4,1)
  M_inv_tau : Gain  Gain=1/p2_tau_m
  M_mix : Gain  Gain=Gamma_mix  Multiplication=Matrix(K*u)
  M_sat : Saturate  UpperLimit=f_max  LowerLimit=0
  M_sel_f : Selector  InputPortWidth=4  IndexOptions=Index vector (dialog)  Indices=1  OutputSizes=1
  M_sel_tau : Selector  InputPortWidth=4  IndexOptions=Index vector (dialog)  Indices=[2 3 4]  OutputSizes=1
  N6_prm : Constant  Value=p2_prm_n6
  N6_s : UnitDelay  InitialCondition=zeros(4,1)  SampleTime=p2_Ts_att  HasFrameUpgradeWarning=on
  N6_z_d : ZeroOrderHold  SampleTime=p2_Ts_att
  N6_z_g : ZeroOrderHold  SampleTime=p2_Ts_att
  N6_z_v : ZeroOrderHold  SampleTime=p2_Ts_att
  N6_z_wm : ZeroOrderHold  SampleTime=p2_Ts_att
  N6_z_ws : ZeroOrderHold  SampleTime=p2_Ts_att
  P2_H3 : MATLAB Function  TreatAsAtomicUnit=on
  P2_H3_out : MATLAB Function  TreatAsAtomicUnit=on
  P2_M3 : MATLAB Function  TreatAsAtomicUnit=on
  P2_N6 : MATLAB Function  TreatAsAtomicUnit=on
  P2_Trans : MATLAB Function  TreatAsAtomicUnit=on
  P2_WindHat : MATLAB Function  TreatAsAtomicUnit=on
  P2_x : Integrator  InitialCondition=[p2_ic_pos(1);p2_ic_pos(2);p2_ic_pos(3); p2_ic_vel(1);p2_ic_vel(2);p2_ic_vel(3); 0;0;-1; 0;0;0]
  S_acc_bias : Constant  Value=p2_bias_acc
  S_acc_noise : RandomNumber  Variance=p2_var_acc  Seed=p2_seed_acc  SampleTime=p2_Ts_att
  S_acc_sum : Sum  Inputs=+++
  S_acc_zoh : ZeroOrderHold  SampleTime=p2_Ts_att
  S_eta_zoh : ZeroOrderHold  SampleTime=p2_Ts_att
  S_gyr_noise : RandomNumber  Variance=p2_var_gyro  Seed=p2_seed_gyro  SampleTime=p2_Ts_att
  S_gyr_sum : Sum
  S_gyr_zoh : ZeroOrderHold  SampleTime=p2_Ts_att
  S_pos_delay : Delay  DelayLength=p2_nd_pos  InitialCondition=[p2_ic_pos(1);p2_ic_pos(2);p2_ic_pos(3)]  SampleTime=p2_Ts_pos
  S_pos_noise : RandomNumber  Variance=p2_var_pos  Seed=p2_seed_pos  SampleTime=p2_Ts_pos
  S_pos_sum : Sum
  S_pos_zoh : ZeroOrderHold  SampleTime=p2_Ts_pos
  S_vel_diff : Sum  Inputs=+-
  S_vel_gain : Gain  Gain=1/p2_Ts_pos
  S_vel_prev : UnitDelay  InitialCondition=[p2_ic_pos(1);p2_ic_pos(2);p2_ic_pos(3)] - [p2_ic_vel(1);p2_ic_vel(2);p2_ic_vel(3)]*p2_Ts_pos  SampleTime=p2_Ts_pos  HasFrameUpgradeWarning=on
  T_gam : Terminator
  T_h3 : Terminator
  T_nu : Terminator
  V_Fcmd_d : VariantSource
  V_acc_d : VariantSource
  V_acc_s : VariantSource
  V_eta_d : VariantSource
  V_fthr_d : VariantSource
  V_gam_d : VariantSource
  V_gam_s : VariantSource
  V_gyr_d : VariantSource
  V_gyr_s : VariantSource
  V_lag : VariantSource
  V_nu_d : VariantSource
  V_nu_s : VariantSource
  V_tau_d : VariantSource
  W_meas : FromWorkspace  VariableName=wind_meas_ts  Interpolate=off  OutputAfterFinalValue=Holding final value
  W_orac : FromWorkspace  VariableName=w_oracle_ts  Interpolate=off  OutputAfterFinalValue=Holding final value
  W_pred : FromWorkspace  VariableName=what_ts  Interpolate=off  OutputAfterFinalValue=Holding final value
  W_sel : MultiPortSwitch  DataPortOrder=Zero-based contiguous  zeroidx=on  SaturateOnIntegerOverflow=off  InputSameDT=off
  W_selc : Constant  Value=wind_use_pred
  W_true : FromWorkspace  VariableName=wind_ts  OutputAfterFinalValue=Holding final value
  X_gam : Selector  InputPortWidth=12  IndexOptions=Index vector (dialog)  Indices=[1 2 3]  OutputSizes=1
  X_nu : Selector  InputPortWidth=12  IndexOptions=Index vector (dialog)  Indices=[4 5 6]  OutputSizes=1
  prm : Constant  Value=p2_prm
  prm_w : Constant  Value=p2_prm_w
  o_gamma : Outport
  o_nu : Outport  Port=2
  o_nu_dot : Outport  Port=3
  o_d_mf : Outport  Port=4
  o_d_lf : Outport  Port=5
  o_tau_plant : Outport  Port=6
  o_gamma_c : Outport  Port=7
  o_nu_c : Outport  Port=8
  o_nu_dot_c : Outport  Port=9
  o_omega_c : Outport  Port=10
  o_eta_c : Outport  Port=11
  o_Fcmd_c : Outport  Port=12
  o_fthr_c : Outport  Port=13
  o_tau_cmd_c : Outport  Port=14
  o_dlf_p2 : Outport  Port=15
  o_dmf_n6 : Outport  Port=16
  o_dmf_h3 : Outport  Port=17
  o_dmf_h4 : Outport  Port=18
  o_dmf_m3n : Outport  Port=19
  o_dmf_m3p : Outport  Port=20
  wires:
  X_gam/1 -> D_pos_zoh/1, S_pos_zoh/1, V_gam_d/2, o_gamma/1
  X_nu/1 -> D_vel_zoh/1, V_nu_d/2, o_nu/1
  P2_H3/1(s_next) -> H3_s/1
  V_acc_s/1 -> H3_z_a/1, o_nu_dot_c/1
  V_eta_d/1 -> H3_z_e/1, o_eta_c/1
  V_fthr_d/1 -> H3_z_f/1, o_fthr_c/1
  [Fcmd] -> H_Fcmd/1, V_Fcmd_d/2
  [fthr] -> H_fthr/1, V_fthr_d/2
  [tau_cmd] -> H_tau_cmd/1, V_tau_d/2
  V_Fcmd_d/1 -> L_Fcmd/1, o_Fcmd_c/1
  V_lag/1 -> L_f/1, M_mix/1
  V_gam_s/1 -> L_gamma_c/1, M3_z_gc/1, o_gamma_c/1
  P2_M3/4(mon) -> L_m3/1
  P2_Trans/7(mon) -> L_mon/1
  P2_N6/3(mon) -> L_n6/1
  S_acc_noise/1 -> L_nacc/1, S_acc_sum/2
  S_gyr_noise/1 -> L_ngyr/1, S_gyr_sum/2
  S_pos_noise/1 -> L_npos/1, S_pos_sum/2
  V_nu_s/1 -> L_nu_c/1, N6_z_v/1, P2_WindHat/2(nu_c), o_nu_c/1
  P2_M3/1(s_next) -> M3_s/1
  [acc_d] -> M3_z_ad/1
  [gamma_d] -> M3_z_gd/1
  [nu_d] -> M3_z_nd/1
  M_sat/1 -> M_err/1, V_lag/2
  M_f/1 -> M_err/2, V_lag/1
  M_inv_tau/1 -> M_f/1
  M_err/1 -> M_inv_tau/1
  [f_i] -> M_sat/1
  M_mix/1 -> M_sel_f/1, M_sel_tau/1
  P2_N6/1(s_next) -> N6_s/1
  [dmf_do] -> N6_z_d/1
  [p2_wgate] -> N6_z_g/1
  W_meas/1 -> N6_z_wm/1, W_sel/2
  W_sel/1 -> N6_z_ws/1, P2_WindHat/1(w)
  H3_s/1 -> P2_H3/1(s), P2_H3_out/1(s)
  H3_z_a/1 -> P2_H3/2(a_meas), P2_M3/8(a_meas)
  H3_z_f/1 -> P2_H3/3(f_cmd)
  H3_z_e/1 -> P2_H3/4(eta)
  H3_prm/1 -> P2_H3/5(prm), P2_H3_out/2(prm)
  M3_s/1 -> P2_M3/1(s)
  N6_z_wm/1 -> P2_M3/2(w_meas), P2_N6/2(w_meas)
  N6_z_v/1 -> P2_M3/3(vQ), P2_N6/4(vQ)
  M3_z_gd/1 -> P2_M3/4(gam_d)
  M3_z_nd/1 -> P2_M3/5(nu_d)
  M3_z_ad/1 -> P2_M3/6(acc_d)
  M3_z_gc/1 -> P2_M3/7(gam_c)
  M3_prm/1 -> P2_M3/9(prm)
  N6_s/1 -> P2_N6/1(s)
  N6_z_ws/1 -> P2_N6/3(w_sig)
  N6_z_d/1 -> P2_N6/5(dmf_do)
  N6_z_g/1 -> P2_N6/6(gate)
  N6_prm/1 -> P2_N6/7(prm)
  P2_x/1 -> P2_Trans/1(x), X_gam/1, X_nu/1
  M_sel_f/1 -> P2_Trans/2(f_act)
  [eta] -> P2_Trans/3(eta), S_eta_zoh/1, V_eta_d/2
  W_true/1 -> P2_Trans/4(w)
  prm/1 -> P2_Trans/5(prm)
  prm_w/1 -> P2_WindHat/3(prm_w)
  P2_Trans/1(dx) -> P2_x/1
  S_acc_zoh/1 -> S_acc_sum/1, V_acc_d/1
  S_acc_bias/1 -> S_acc_sum/3
  P2_Trans/4(a_Q) -> S_acc_zoh/1, V_acc_d/2, o_nu_dot/1
  S_gyr_zoh/1 -> S_gyr_sum/1, V_gyr_d/1
  [omega] -> S_gyr_zoh/1, V_gyr_d/2
  S_pos_zoh/1 -> S_pos_delay/1
  S_pos_delay/1 -> S_pos_sum/1
  S_pos_sum/1 -> S_vel_diff/1, S_vel_prev/1, V_gam_s/1
  S_vel_prev/1 -> S_vel_diff/2
  S_vel_diff/1 -> S_vel_gain/1
  P2_Trans/2(gam) -> T_gam/1
  P2_H3/2(d_hat) -> T_h3/1
  P2_Trans/3(nu) -> T_nu/1
  H_Fcmd/1 -> V_Fcmd_d/1
  S_acc_sum/1 -> V_acc_s/1
  V_acc_d/1 -> V_acc_s/2
  S_eta_zoh/1 -> V_eta_d/1
  H_fthr/1 -> V_fthr_d/1
  D_pos_zoh/1 -> V_gam_d/1
  V_gam_d/1 -> V_gam_s/2
  S_gyr_sum/1 -> V_gyr_s/1
  V_gyr_d/1 -> V_gyr_s/2
  D_vel_zoh/1 -> V_nu_d/1
  S_vel_gain/1 -> V_nu_s/1
  V_nu_d/1 -> V_nu_s/2
  H_tau_cmd/1 -> V_tau_d/1
  W_selc/1 -> W_sel/1
  W_pred/1 -> W_sel/3
  W_orac/1 -> W_sel/4
  P2_Trans/5(d_mf) -> o_d_mf/1
  P2_Trans/6(d_lf) -> o_d_lf/1
  M_sel_tau/1 -> o_tau_plant/1
  V_gyr_s/1 -> o_omega_c/1
  V_tau_d/1 -> o_tau_cmd_c/1
  P2_WindHat/1(dlf_hat) -> o_dlf_p2/1
  P2_N6/2(delta) -> o_dmf_n6/1
  P2_H3_out/1(d_hat) -> o_dmf_h3/1
  H4_off/1 -> o_dmf_h4/1
  P2_M3/2(dM_now) -> o_dmf_m3n/1
  P2_M3/3(dM_pred) -> o_dmf_m3p/1

== matlab function baseline1/UAV_Plant/Trans_4a ==
  data: F_act input; nu_dot output; d_mf input; d_lf input; m input; g input
function nu_dot = translational_dynamics(F_act, d_mf, d_lf, m, g)
%#codegen
% --- Khai bao kich thuoc output (de Simulink suy dung kich thuoc tin hieu) ---
nu_dot = zeros(3,1);
% Dong luc hoc tinh tien, pt. (4a)/(7) Guo 2020:
%   m*nu_dot = F - m*g*e3 + d_mf + d_lf
nu_dot = (F_act - m*g*[0;0;1] + d_mf + d_lf)/m;
end

== matlab function baseline1/UAV_Plant/Rot_5 ==
  data: tau_act input; eta_ddot output; d_ltau input; eta input; eta_dot input; Ixx input; Iyy input; Izz input
function eta_ddot = rotational_dynamics(tau_act, d_ltau, eta, eta_dot, Ixx, Iyy, Izz)
%#codegen
% --- Khai bao kich thuoc output (de Simulink suy dung kich thuoc tin hieu) ---
eta_ddot = zeros(3,1);
% Dong luc hoc quay, pt. (5)/(7) Guo 2020 (Lagrange-Euler, toa do eta):
%   M(eta)*eta_ddot + C(eta,eta_dot)*eta_dot = tau + d_ltau
% M, C nguyen van trang 3 bai bao (Raffo et al. 2010).
M = M_of_eta(eta, Ixx, Iyy, Izz);
C = C_of_eta(eta, eta_dot, Ixx, Iyy, Izz);
eta_ddot = M \ (tau_act + d_ltau - C*eta_dot);
end

function M = M_of_eta(eta, Ixx, Iyy, Izz)
phi = eta(1); theta = eta(2);
cphi = cos(phi); sphi = sin(phi);
cth  = cos(theta); sth = sin(theta);
M = [Ixx,       0,                        -Ixx*sth;
     0,         Iyy*cphi^2 + Izz*sphi^2,  (Iyy-Izz)*cphi*sphi*cth;
     -Ixx*sth, (Iyy-Izz)*cphi*sphi*cth,   Ixx*sth^2 + (Iyy*sphi^2 + Izz*cphi^2)*cth^2];
end

function C = C_of_eta(eta, eta_dot, Ixx, Iyy, Izz)
phi = eta(1); theta = eta(2);
phid = eta_dot(1); thetad = eta_dot(2); psid = eta_dot(3);
cphi = cos(phi); sphi = sin(phi);
cth  = cos(theta); sth = sin(theta);
c11 = 0;
c12 = (Iyy-Izz)*(thetad*cphi*sphi + psid*sphi^2*cth) ...
      - (Ixx + Iyy*cphi^2 - Izz*cphi^2)*psid*cth;
c13 = (Izz-Iyy)*psid*cphi*sphi*cth^2;
c21 = (Izz-Iyy)*(thetad*cphi*sphi + psid*sphi^2*cth) ...
      + (Ixx + Iyy*cphi^2 - Izz*cphi^2)*psid*cth;
c22 = (Izz-Iyy)*phid*cphi*sphi;
c23 = (-Ixx + Iyy*sphi^2 + Izz*cphi^2)*psid*sth*cth;
c31 = (Iyy-Izz)*psid*cth^2*sphi*cphi - Ixx*thetad*cth;
c32 = (Izz-Iyy)*(thetad*cphi*sphi*sth + phid*sphi^2*cth - phid*cphi^2*cth) ...
      + (Ixx - Iyy*sphi^2 - Izz*cphi^2)*psid*sth*cth;
c33 = (Iyy-Izz)*phid*cphi*sphi*cth^2 ...
      + (Ixx - Iyy*sphi^2 - Izz*cphi^2)*thetad*cth*sth;
C = [c11 c12 c13; c21 c22 c23; c31 c32 c33];
end

== matlab function baseline1/UAV_Plant/Body_Rates ==
  data: eta input; omega output; eta_dot input
function omega = euler_to_body_rates(eta, eta_dot)
%#codegen
% --- Khai bao kich thuoc output (de Simulink suy dung kich thuoc tin hieu) ---
omega = zeros(3,1);
% omega = T(eta)*eta_dot: doi Euler rates (world) sang body rates cho (18).
phi = eta(1); theta = eta(2);
cphi = cos(phi); sphi = sin(phi);
cth  = cos(theta); sth = sin(theta);
T = [1, 0,    -sth;
     0, cphi,  sphi*cth;
     0, -sphi, cphi*cth];
omega = T*eta_dot;
end

== matlab function baseline1/Position_Observers/DO_12 ==
  data: gamma input; z_dot output; nu input; z input; F input; dlf_hat input; A_do input; B_do input; l_gain input; G_do input; g input
function z_dot = do_derivative(gamma, nu, z, F, dlf_hat, A_do, B_do, l_gain, G_do, g)
%#codegen
% --- Khai bao kich thuoc output (de Simulink suy dung kich thuoc tin hieu) ---
z_dot = zeros(size(z));   % kich thuoc theo z: 6 trang thai (hoa 1) hoac 12 (hoa [1 3])
% Disturbance Observer, pt. (11)-(13) Guo 2020 (l chon hang so, Sec. 3.3.1):
%   p(gamma,nu) = l*[gamma; nu]                                      (11b,13)
%   xi_hat  = z + p                                                   (11a)
%   dmf_hat = B*xi_hat                                                (12)
%   z_dot   = (A - l*G*B)*z + A*p - l*(G*B*p + f(nu) + G*F + G*dlf_hat) (12)
% voi f(nu) = [nu; 0; 0; -g].
% F o day la wrench THUC da ap (F_act) - phan mem onboard biet chinh xac
% (bao hoa nam trong code, eta do duoc) -> uoc luong khong lan artifact.
% (dmf_hat = B*(z+p) duoc tinh o khoi DO_Out rieng - pha algebraic loop)
p    = l_gain*[gamma; nu];
f_nu    = [nu; 0; 0; -g];
z_dot   = (A_do - l_gain*G_do*B_do)*z + A_do*p ...
          - l_gain*(G_do*B_do*p + f_nu + G_do*F + G_do*dlf_hat);
end

== matlab function baseline1/Position_Observers/DO_Out ==
  data: gamma input; dmf_hat output; nu input; z input; B_do input; l_gain input
function dmf_hat = do_output(gamma, nu, z, B_do, l_gain)
%#codegen
% --- Khai bao kich thuoc output (de Simulink suy dung kich thuoc tin hieu) ---
dmf_hat = zeros(3,1);
% Dau ra DO, pt. (11a) + dong cuoi (12) Guo 2020:
%   xi_hat  = z + p(gamma,nu),  p = l*[gamma; nu]
%   dmf_hat = B*xi_hat
% Tach rieng khoi nay (khong nhan F) de pha algebraic loop: uoc luong chi
% phu thuoc TRANG THAI (z, gamma, nu), dung ban chat toan hoc cua DO.
dmf_hat = B_do*(z + l_gain*[gamma; nu]);
end

== matlab function baseline1/Position_Observers/ESO_15 ==
  data: gamma input; zp_dot output; zp input; F input; dmf_hat input; Kp1 input; Kp2 input; Kp3 input; m input; g input
function zp_dot = eso_pos_derivative(gamma, zp, F, dmf_hat, Kp1, Kp2, Kp3, m, g)
%#codegen
% --- Khai bao kich thuoc output (de Simulink suy dung kich thuoc tin hieu) ---
zp_dot = zeros(9,1);
% ESO vong vi tri, pt. (14)-(15) Guo 2020. Trang thai zp = [zp1;zp2;zp3]:
%   zp1_dot = zp2 + Kp1*ep1
%   zp2_dot = (1/m)*(F - m*g*e3 + zp3 + dmf_hat) + Kp2*ep1
%   zp3_dot = Kp3*ep1,     ep1 = gamma - zp1
% dlf_hat = zp3 (uoc luong nhieu gio/derivative-bounded).
zp1 = zp(1:3); zp2 = zp(4:6); zp3 = zp(7:9);
ep1 = gamma - zp1;
zp1_dot = zp2 + Kp1*ep1;
zp2_dot = (1/m)*(F - m*g*[0;0;1] + zp3 + dmf_hat) + Kp2*ep1;
zp3_dot = Kp3*ep1;
zp_dot  = [zp1_dot; zp2_dot; zp3_dot];
% (dlf_hat = zp3 duoc lay o khoi ESO_Out rieng - pha algebraic loop)
end

== matlab function baseline1/Position_Observers/ESO_Out ==
  data: zp input; dlf_hat output
function dlf_hat = eso_pos_output(zp)
%#codegen
% --- Khai bao kich thuoc output (de Simulink suy dung kich thuoc tin hieu) ---
dlf_hat = zeros(3,1);
% Dau ra ESO vi tri, pt. (15): dlf_hat = zp3 (uoc luong nhieu gio).
% Tach rieng (chi phu thuoc trang thai zp) de pha algebraic loop.
dlf_hat = zp(7:9);
end

== matlab function baseline1/Attitude_Observer/ESO_att_20 ==
  data: eta input; za_dot output; za input; tau input; Ka1 input; Ka2 input; Ka3 input; Ixx input; Iyy input; Izz input
function za_dot = eso_att_derivative(eta, za, tau, Ka1, Ka2, Ka3, Ixx, Iyy, Izz)
%#codegen
% --- Khai bao kich thuoc output (de Simulink suy dung kich thuoc tin hieu) ---
za_dot = zeros(9,1);
% ESO vong tu the theo pt. (19)-(20) Guo 2020, cai dat DAY DU M_hat, C_hat
% tinh tu uoc luong (za1, za2) - khong luoc bo C.
% *** DANG CHUAN HOA (Remark trong paper cua ban) ***
% Neu za3 uoc luong truc tiep d_ltau (N.m) va ap nguyen gain Appendix
% Ka3 = 3906*I3, da thuc dac trung moi truc la s^3+50s^2+833s+3906/I_ii;
% voi I_xx = 0.01: 50*833 = 41650 < 390600 -> MAT on dinh (Routh).
% Bo gain Appendix khop chinh xac bandwidth parameterization (s+w0)^3
% (3w0 = 50, 3w0^2 = 833 -> w0 ~ 16.7 rad/s) => nhom tac gia tham so hoa
% theo NHIEU GIA TOC GOC. Do do:
%   za3 := uoc luong M^-1*d_ltau  (rad/s^2)
%   za2_dot = M_hat\(tau - C_hat*za2) + za3 + Ka2*ea1
% -> da thuc moi truc: s^3 + 50 s^2 + 833 s + 3906 (on dinh, dung Appendix).
% Quy doi ve moment o khoi Att_Dist_Output: dltau_hat = M(za1)*za3.
za1 = za(1:3); za2 = za(4:6); za3 = za(7:9);
ea1 = eta - za1;
Mhat = M_of_eta(za1, Ixx, Iyy, Izz);
Chat = C_of_eta(za1, za2, Ixx, Iyy, Izz);
za_dot = [za2 + Ka1*ea1;
          Mhat\(tau - Chat*za2) + za3 + Ka2*ea1;
          Ka3*ea1];
end

function M = M_of_eta(eta, Ixx, Iyy, Izz)
phi = eta(1); theta = eta(2);
cphi = cos(phi); sphi = sin(phi);
cth  = cos(theta); sth = sin(theta);
M = [Ixx,       0,                        -Ixx*sth;
     0,         Iyy*cphi^2 + Izz*sphi^2,  (Iyy-Izz)*cphi*sphi*cth;
     -Ixx*sth, (Iyy-Izz)*cphi*sphi*cth,   Ixx*sth^2 + (Iyy*sphi^2 + Izz*cphi^2)*cth^2];
end

function C = C_of_eta(eta, eta_dot, Ixx, Iyy, Izz)
phi = eta(1); theta = eta(2);
phid = eta_dot(1); thetad = eta_dot(2); psid = eta_dot(3);
cphi = cos(phi); sphi = sin(phi);
cth  = cos(theta); sth = sin(theta);
c11 = 0;
c12 = (Iyy-Izz)*(thetad*cphi*sphi + psid*sphi^2*cth) ...
      - (Ixx + Iyy*cphi^2 - Izz*cphi^2)*psid*cth;
c13 = (Izz-Iyy)*psid*cphi*sphi*cth^2;
c21 = (Izz-Iyy)*(thetad*cphi*sphi + psid*sphi^2*cth) ...
      + (Ixx + Iyy*cphi^2 - Izz*cphi^2)*psid*cth;
c22 = (Izz-Iyy)*phid*cphi*sphi;
c23 = (-Ixx + Iyy*sphi^2 + Izz*cphi^2)*psid*sth*cth;
c31 = (Iyy-Izz)*psid*cth^2*sphi*cphi - Ixx*thetad*cth;
c32 = (Izz-Iyy)*(thetad*cphi*sphi*sth + phid*sphi^2*cth - phid*cphi^2*cth) ...
      + (Ixx - Iyy*sphi^2 - Izz*cphi^2)*psid*sth*cth;
c33 = (Iyy-Izz)*phid*cphi*sphi*cth^2 ...
      + (Ixx - Iyy*sphi^2 - Izz*cphi^2)*thetad*cth*sth;
C = [c11 c12 c13; c21 c22 c23; c31 c32 c33];
end

== matlab function baseline1/Attitude_Observer/Att_Dist_Out ==
  data: za input; dltau_hat output; Ixx input; Iyy input; Izz input
function dltau_hat = att_disturbance_output(za, Ixx, Iyy, Izz)
%#codegen
% --- Khai bao kich thuoc output (de Simulink suy dung kich thuoc tin hieu) ---
dltau_hat = zeros(3,1);
% Quy doi uoc luong nhieu gia toc goc (za3) ve nhieu MOMENT cho luat (18):
%   dltau_hat = M(za1)*za3   (N.m)
phi = za(1); theta = za(2);
cphi = cos(phi); sphi = sin(phi);
cth  = cos(theta); sth = sin(theta);
M = [Ixx,       0,                        -Ixx*sth;
     0,         Iyy*cphi^2 + Izz*sphi^2,  (Iyy-Izz)*cphi*sphi*cth;
     -Ixx*sth, (Iyy-Izz)*cphi*sphi*cth,   Ixx*sth^2 + (Iyy*sphi^2 + Izz*cphi^2)*cth^2];
dltau_hat = M*za(7:9);
end

== matlab function baseline1/Disturbances/Dist_Gen ==
  data: t input; d_mf_sin output size=[3 1]; payload_amp input; payload_sigma input; wind_amp input; d_lf output size=[3 1]; d_ltau output size=[3 1]
function [d_mf_sin, d_lf, d_ltau] = disturbance_generator(t, payload_amp, payload_sigma, wind_amp)
%#codegen
%DISTURBANCE_GENERATOR  Nguon nhieu ngoai cua Test 4.
%
%  d_mf_sin : nhieu tai, luc, he quan tinh          [N]     pt. (6)
%  d_lf     : luc gio, hang so trong he the gioi    [N]
%  d_ltau   : nhieu moment ngoai                    [N.m]   -- KHONG MO HINH HOA
%
%  ----------------------------------------------------------------------
%  VE d_ltau
%  ----------------------------------------------------------------------
%  Guo et al. 2020 co Assumption 3 cho nhieu moment, nhung KHONG cong bo dang
%  song, bien do, hay huong cua no. Bom vao mot dang song tu nghi ra la them
%  mot bac tu do khong ai kiem chung duoc, va no se di thang vao bang ket qua
%  duoi danh nghia "tai lap".
%
%  Nen d_ltau = 0, va do la mot LUA CHON CO CHU DICH phai khai bao trong paper:
%  pham vi cua ban la nhieu LUC (tai + gio), khong phai nhieu MOMENT.
%
%  He qua phai noi ro: ESO tu the trong cau hinh ESO/MOBADC khong co nhieu
%  ngoai nao de khu. No van lam viec (khu sai lech mo hinh va ghep truc), nhung
%  bat ky phat bieu nao ve kha nang khang nhieu MOMENT deu khong duoc thi
%  nghiem nay chong do.
%
%  Ban truoc co mot doi so amp_tau o day ma than ham khong dung den, trong khi
%  init khai bao 0.05 N.m va ca hai run script in no ra tieu de bang. Bang khi
%  do dang bao cao mot dieu kien thi nghiem khong ton tai.
%  Xem docs/AUDIT.md muc A1.

d_mf_sin = zeros(3,1); d_lf = zeros(3,1); d_ltau = zeros(3,1);

d_mf_sin = [0; payload_amp*sin(payload_sigma*t); 0];

psi_w = 40*pi/180;                       % [PAPER Fig. 8b] huong gio NE 40 deg
d_lf  = wind_amp*[cos(psi_w); sin(psi_w); 0];

d_ltau = zeros(3,1);                     % khong mo hinh hoa - xem chu thich
end

== matlab function baseline1/Translational_Control/Pos_Ctrl_9 ==
  data: gamma_d input; F output; nu_d input; acc_d input; gamma input; nu input; dmf_hat input; dlf_hat input; Kgamma input; Knu input; m input; g input
function F = position_controller(gamma_d, nu_d, acc_d, gamma, nu, dmf_hat, dlf_hat, Kgamma, Knu, m, g)
%#codegen
% --- Khai bao kich thuoc output (de Simulink suy dung kich thuoc tin hieu) ---
F = zeros(3,1);
% Luat dieu khien vong vi tri, pt. (8)-(9) Guo 2020:
%   e_gamma = gamma_d - gamma;  e_nu = nu_d - nu                      (8)
%   a_d = Kgamma*e_gamma + Knu*e_nu + g*e3 + gamma_ddot_d             (9)
%   F   = m*a_d - dmf_hat - dlf_hat                                   (9)
% PID mode (Remark 9): dmf_hat = dlf_hat = 0 (qua Manual Switch).
e_gamma = gamma_d - gamma;
e_nu    = nu_d    - nu;
a_d = Kgamma*e_gamma + Knu*e_nu + g*[0;0;1] + acc_d;
F   = m*a_d - dmf_hat - dlf_hat;
end

== matlab function baseline1/Logging_Metrics/Err_Norm ==
  data: gamma input; err output; gamma_d input
function err = error_norm(gamma, gamma_d)
%#codegen
% --- Khai bao kich thuoc output (de Simulink suy dung kich thuoc tin hieu) ---
err = 0;
% Sai so vi tri tuc thoi ||gamma - gamma_d|| (dinh nghia Table 1 bai bao).
err = norm(gamma - gamma_d);
end

== matlab function baseline1/Disturbances/Payload_Pendulum/pend_deriv ==
  data: xp input; xp_dot output; a_uav input; F_wp input; m_p input; L input; zeta_p input; g input
function xp_dot = payload_pendulum_derivative(xp, a_uav, F_wp, m_p, L, zeta_p, g)
%#codegen
%PAYLOAD_PENDULUM_DERIVATIVE  Dong luc hoc con lac treo duoi UAV.
%
%  Paste noi dung file nay vao mot khoi MATLAB Function trong Simulink.
%
%  Trang thai  xp = [th_x; thd_x; th_y; thd_y]     (rad, rad/s)
%  Vao
%     a_uav : 2x1  gia toc NGANG cua UAV, he QUAN TINH        [m/s^2]
%             -> lay tu nu_dot(1:2), QUA MOT KHOI MEMORY (xem WIRING.md)
%     F_wp  : 2x1  luc gio tac dung TRUC TIEP len tai          [N]
%             -> Giai doan 2.1 noi Constant [0;0] vao day.
%                Cong da co san de Giai doan 2.2 cam vao khong phai sua khoi.
%     m_p, L, zeta_p, g : tham so (tu init_MOBADC_params)
%
%  Phuong trinh, moi truc (con lac phang, day cung, khoi luong tap trung):
%
%     thddot = -(g/L) sin(th) - (a/L) cos(th)
%              - 2 zeta wn thdot + F_w/(m_p L),      wn = sqrt(g/L)
%
%  Hai truc coi nhu doc lap.  Con lac cau that co so hang ghep bac
%  th^2*thdot, rat nho o bien do lac o day nhung KHAC KHONG - do la mot
%  thanh phan cua residual, phai ghi vao bai chu khong phai bo qua im lang.
%
%  KHONG dung khoi nay de dat dieu kien dau: Integrator ngoai giu state,
%  IC = [0;0;0;0].

xp_dot = zeros(4,1);

wn = sqrt(g/L);
for k = 0:1
    th  = xp(2*k + 1);
    thd = xp(2*k + 2);

    xp_dot(2*k + 1) = thd;
    xp_dot(2*k + 2) = -(g/L)*sin(th) - (a_uav(k+1)/L)*cos(th) ...
                      - 2*zeta_p*wn*thd + F_wp(k+1)/(m_p*L);
end
end
